simulink model "Force_Control"  (R2020b)
settings: Solver=VariableStepAuto  StartTime=0.0  StopTime=20  RelTol=1e-3
values from neighbouring files (symbols this model uses):
  B = myRobot.B_Lagrangian    [hw14_main.m]
  C = myRobot.C_Lagrangian    [hw14_main.m]
  dJ = dJ(1:3  ,:)    [hw14_main.m]
  F = myRobot.F    [hw14_main.m]
  fd = [0;1;0]    [hw14_main.m]
  G = myRobot.G_Lagrangian    [hw14_main.m]
  J_inv = pinv(J)    [hw14_main.m]
  Ja = Ja(1:3,:)    [hw14_main.m]
  K = diag([1 1 1])    [hw14_main.m]
  Kd = diag([1 20 1])    [hw14_main.m]
  Kf = diag([1 10 1]).*10    [hw14_main.m]
  Ki = diag([1 10 1])    [hw14_main.m]
  Kp = diag([1 0.5 1])    [hw14_main.m]
  Md = diag([1 1 1])    [hw14_main.m]
  Md_inv = pinv(Md)    [hw14_main.m]
  xr = [0;0.3;0]    [hw14_main.m]
settings Model: Creator=nicol  LastModifiedBy=nicol

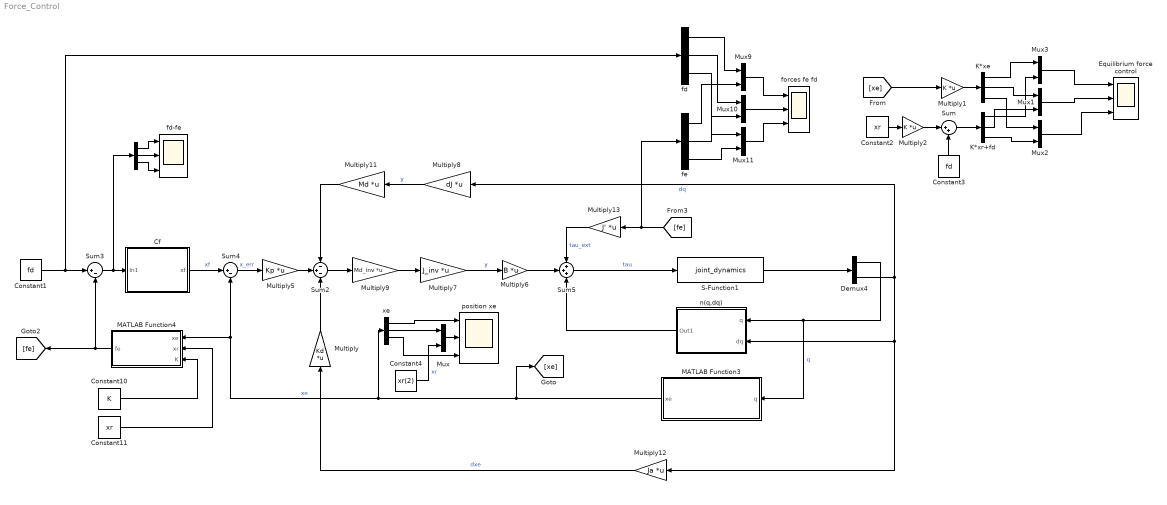
== system Force_Control ==
  " " : Demux  Outputs=3
  " fd-fe " : Scope  NumInputPorts=3
  Cf : Subsystem
  Constant1 : Constant  Value=fd
  Constant10 : Constant  Value=K
  Constant11 : Constant  Value=xr
  Constant2 : Constant  Value=xr
  Constant3 : Constant  Value=fd
  Constant4 : Constant  Value=xr(2)
  Demux4 : Demux  Outputs=2
  Equilibrium force control : Scope  NumInputPorts=3
  K*xe : Demux  Outputs=3
  K*xr+fd : Demux  Outputs=3
  MATLAB Function3 : MATLAB Function  TreatAsAtomicUnit=on
  MATLAB Function4 : MATLAB Function  TreatAsAtomicUnit=on
  Multiply : Gain  Gain=Kd  Multiplication=Matrix(K*u)
  Multiply1 : Gain  Gain=K  Multiplication=Matrix(K*u)
  Multiply11 : Gain  Gain=Md  Multiplication=Matrix(K*u)
  Multiply12 : Gain  Gain=Ja  Multiplication=Matrix(K*u)
  Multiply13 : Gain  Gain=J'  Multiplication=Matrix(K*u)
  Multiply2 : Gain  Gain=K  Multiplication=Matrix(K*u)
  Multiply5 : Gain  Gain=Kp  Multiplication=Matrix(K*u)
  Multiply6 : Gain  Gain=B  Multiplication=Matrix(K*u)
  Multiply7 : Gain  Gain=J_inv  Multiplication=Matrix(K*u)
  Multiply8 : Gain  Gain=dJ  Multiplication=Matrix(K*u)
  Multiply9 : Gain  Gain=Md_inv  Multiplication=Matrix(K*u)
  Mux{,1..3,9..11} (7 alike) : Mux  Inputs=2
  S-Function1 : S-Function  FunctionName=joint_dynamics  Parameters=myRobot  SFunctionDeploymentMode=off  EnableBusSupport=off
  Sum : Sum  Inputs=|++
  Sum2 : Sum  Inputs=-+-
  Sum3 : Sum  Inputs=|+-
  Sum4 : Sum  Inputs=|+-
  Sum5 : Sum  Inputs=+++
  fd : Demux  Outputs=3
  fe : Demux  Outputs=3
  forces fe fd : Scope  NumInputPorts=3
  n(q,dq) : Subsystem
  position xe : Scope  NumInputPorts=3
  xe : Demux  Outputs=3
  wires:
  Sum4/1 -> Multiply5/1  "x_err"
  Multiply/1 -> Sum2/3
  Sum2/1 -> Multiply9/1
  Multiply6/1 -> Sum5/2
  Multiply5/1 -> Sum2/2
  Multiply7/1 -> Multiply6/1  "y"
  Multiply11/1 -> Sum2/1
  Multiply8/1 -> Multiply11/1  "y"
  Multiply9/1 -> Multiply7/1
  Sum5/1 -> S-Function1/1  "tau"
  n(q,dq)/1(Out1) -> Sum5/3
  Demux4/2 -> Multiply8/1, Multiply12/1, n(q,dq)/2(dq)  "dq"
  S-Function1/1 -> Demux4/1
  Multiply12/1 -> Multiply/1  "dxe"
  MATLAB Function3/1(xe) -> [xe], Sum4/2, MATLAB Function4/1(xe), xe/1  "xe"
  Constant1/1 -> fd/1, Sum3/1
  MATLAB Function4/1(fe) -> [fe], Sum3/2
  Constant11/1 -> MATLAB Function4/2(xr)
  Constant10/1 -> MATLAB Function4/3(K)
  Demux4/1 -> MATLAB Function3/1(q), n(q,dq)/1(q)  "q"
  Multiply13/1 -> Sum5/1  "tau_ext"
  Cf/1(xf) -> Sum4/1  "xf"
  [fe] -> fe/1, Multiply13/1
  Mux9/1 -> forces fe fd/1
  Mux11/1 -> forces fe fd/3
  fd/2 -> Mux10/1
  Mux10/1 -> forces fe fd/2
  fe/2 -> Mux10/2
  fe/1 -> Mux9/2
  fd/3 -> Mux11/1
  fe/3 -> Mux11/2
  fd/1 -> Mux9/1
  xe/2 -> Mux/1
  xe/3 -> position xe/3
  xe/1 -> position xe/1
  " "/1 -> " fd-fe "/1
  " "/3 -> " fd-fe "/3
  " "/2 -> " fd-fe "/2
  Sum3/1 -> " "/1, Cf/1(In1)
  Constant2/1 -> Multiply2/1
  Constant3/1 -> Sum/2
  [xe] -> Multiply1/1
  Multiply1/1 -> K*xe/1
  Sum/1 -> K*xr+fd/1
  Multiply2/1 -> Sum/1
  K*xe/1 -> Mux3/1
  K*xe/2 -> Mux1/1
  K*xr+fd/1 -> Mux3/2
  K*xe/3 -> Mux2/1
  K*xr+fd/2 -> Mux1/2
  K*xr+fd/3 -> Mux2/2
  Mux3/1 -> Equilibrium force control/1
  Mux1/1 -> Equilibrium force control/2
  Mux2/1 -> Equilibrium force control/3
  Constant4/1 -> Mux/2  "xr"
  Mux/1 -> position xe/2

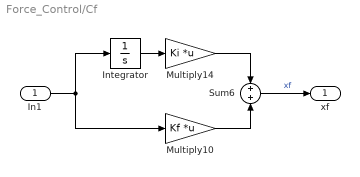
== system Force_Control/Cf ==
  In1 : Inport
  Integrator : Integrator
  Multiply10 : Gain  Gain=Kf  Multiplication=Matrix(K*u)
  Multiply14 : Gain  Gain=Ki  Multiplication=Matrix(K*u)
  Sum6 : Sum
  xf : Outport
  wires:
  Multiply14/1 -> Sum6/1
  Integrator/1 -> Multiply14/1
  In1/1 -> Integrator/1, Multiply10/1
  Multiply10/1 -> Sum6/2
  Sum6/1 -> xf/1  "xf"

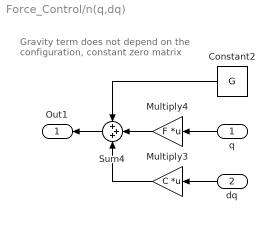
== system Force_Control/n(q,dq) ==
  note: Gravity term does not depend on the
      |  configuration, constant zero matrix
  q : Inport
  dq : Inport  Port=2
  Constant2 : Constant  Value=G  VectorParams1D=off
  Multiply3 : Gain  Gain=C  Multiplication=Matrix(K*u)
  Multiply4 : Gain  Gain=F  Multiplication=Matrix(K*u)
  Sum4 : Sum  Inputs=+++
  Out1 : Outport
  wires:
  Sum4/1 -> Out1/1
  Multiply3/1 -> Sum4/3
  Multiply4/1 -> Sum4/2
  Constant2/1 -> Sum4/1
  q/1 -> Multiply4/1
  dq/1 -> Multiply3/1

== matlab function Force_Control/MATLAB Function4 ==
  data: xe input; fe output; xr input; K input
function fe = getFe(xe,xr,K)
if(xe(2,1)-xr(2,1)>0)
    fe=K*(xe-xr);
    fe(1)=0;
    fe(3)=0;
else
    fe=zeros(3,1);
end

== matlab function Force_Control/MATLAB Function3 ==
  data: q input size=3; xe output size=3
function xe = directKinematics(q)
xe=[ q(1) + 1/5;
    q(3) + 1/5;
    q(2) + 1251/5000]
end
